simulink model "model1"  (R2021b)
settings: Solver=VariableStepAuto  StartTime=0.0  StopTime=10.0  FixedStep=0.001  RelTol=1e-3
undefined symbols (not defined in the file): Newton, Raphson
libraries: simulink x21, slpidlib x7
(part 1 of 2)
settings Model: Creator=O  LastModifiedBy=wangzixuan

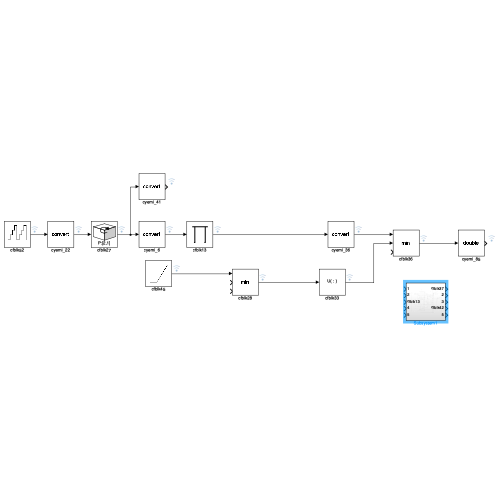
[thumbnail: Simulink's stored preview of the top-level diagram]
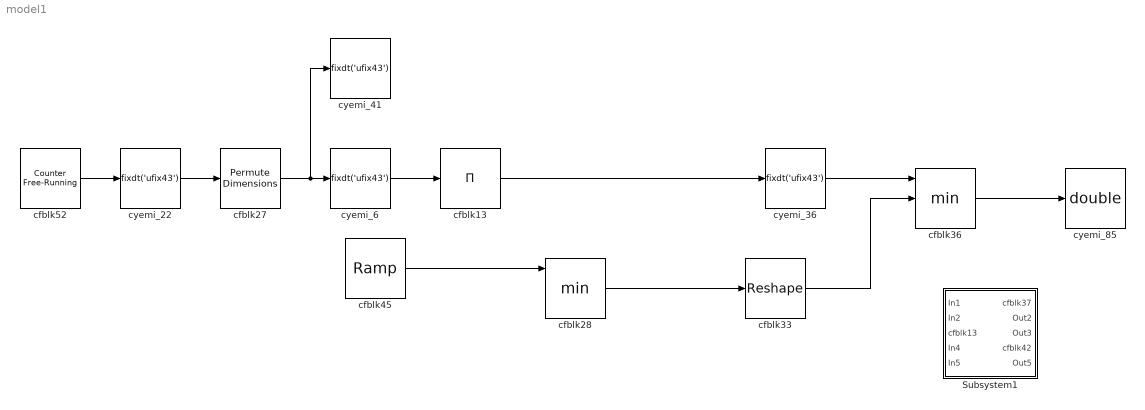
== system model1 ==
  Subsystem1 : Subsystem
  cfblk13 : Product  Inputs=*  OutDataTypeStr=fixdt('ufix43')
  cfblk27 : PermuteDimensions
  cfblk28 : MinMax  Inputs=3  OutDataTypeStr=double
  cfblk33 : Reshape
  cfblk36 : MinMax  Inputs=3  OutDataTypeStr=double
  cfblk45 : simulink/Sources/Ramp  slope=[2140.187855]  start=[6.196724]  InitialOutput=[541750.410278]
  cfblk52 : simulink/Sources/Counter Free-Running  NumBits=[43.000000]  tsamp=1
  cyemi_{6,22,36,41} (4 alike) : DataTypeConversion  OutDataTypeStr=fixdt('ufix43')
  cyemi_85 : DataTypeConversion  OutDataTypeStr=double
  wires:
  cfblk27/1 -> cyemi_41/1, cyemi_6/1
  cfblk52/1 -> cyemi_22/1
  cfblk33/1 -> cfblk36/2
  cyemi_36/1 -> cfblk36/1
  cfblk45/1 -> cfblk28/1
  cfblk36/1 -> cyemi_85/1
  cfblk28/1 -> cfblk33/1
  cyemi_6/1 -> cfblk13/1
  cfblk13/1 -> cyemi_36/1
  cyemi_22/1 -> cfblk27/1

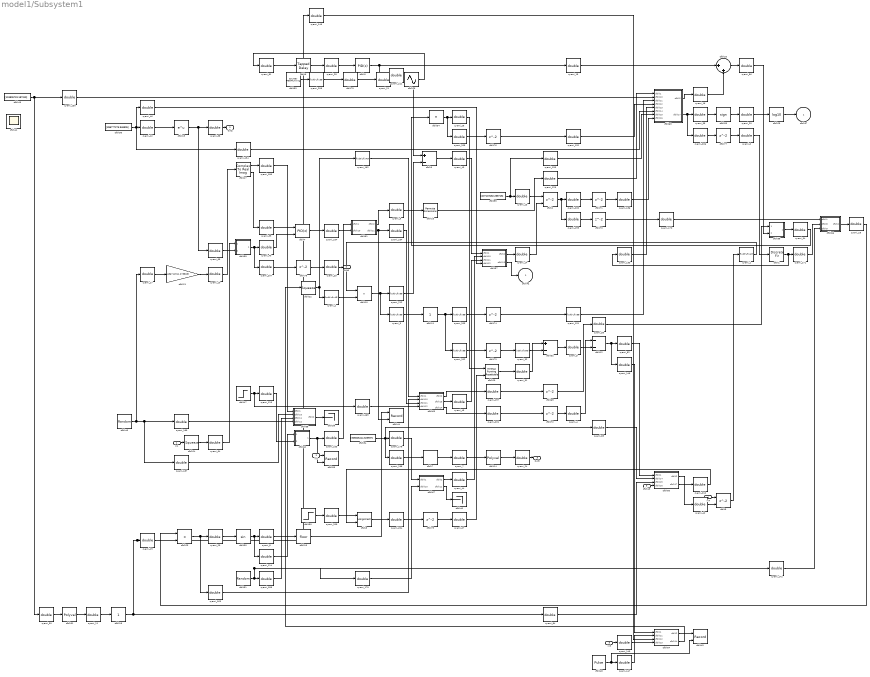
== system model1/Subsystem1 ==
  In1 : Inport
  In2 : Inport  Port=2
  cfblk13 : Inport  Port=3
  In4 : Inport  Port=4
  In5 : Inport  Port=5
  cfblk1 : DiscreteFir  SampleTime=1
  cfblk10 : DotProduct  OutDataTypeStr=fixdt('ufix86')  InputSameDT=on
  cfblk11 : simulink/Math Operations/Slider Gain  gain=1  low=0  high=2
  cfblk12 : Sum  Inputs=--  OutDataTypeStr=double
  cfblk14 : Polyval  Coefs=[ +2.081618890e-019, -1.441693666e-014, +4.719686976e-010, -8.536869453e-006, +1.621573104e-001, -8.087801117e+001 ]
  cfblk15 : Rounding
  cfblk16 : PermuteDimensions
  cfblk17 : ComplexToRealImag
  cfblk18 : simulink/Math Operations/Slider Gain  gain=1  low=0  high=2
  cfblk19 : Math  OutDataTypeStr=double  SaturateOnIntegerOverflow=on
  cfblk2 : Delay  ShowEnablePort=on  SampleTime=1
      settings: InputPortMap=u0,e6
  cfblk20 : Sum  Inputs=|++  OutDataTypeStr=double
  cfblk21 : Gain  Gain=[486711511.278808]  OutDataTypeStr=double
  cfblk22 : Squeeze
  cfblk23 : Product  OutDataTypeStr=double
  cfblk24 : Squeeze
  cfblk25 : Math  Operator=log10  OutDataTypeStr=double  SaturateOnIntegerOverflow=on
  cfblk26 : Sin  TimeSource=Use external signal  SampleTime=0
  cfblk29 : simulink/Math Operations/MinMax Running Resettable  Function=min  vinit=0.0
  cfblk3 : slpidlib/PID Controller  Controller=PID  Form=Parallel  TimeDomain=Discrete-time  UseExternalTs=off  SampleTime=1  IntegratorMethod=Forward Euler  FilterMethod=Forward Euler  ControllerParametersSource=internal  P=1  I=1  D=0  UseFilter=on  N=100  TunerSelectOption=Transfer Function Based (PID Tuner App)  InitialConditionSource=internal  InitialConditionForIntegrator=0  InitialConditionForFilter=0  DifferentiatorICPrevScaledInput=0  ExternalReset=none  TrackingMode=off  Kt=1  LimitOutput=off  SatLimitsSource=internal  UpperSaturationLimit=inf  LowerSaturationLimit=-inf  LinearizeAsGain=off  AntiWindupMode=none  Kb=1  POutMin=[]  POutMax=[]  IOutMin=[]  IOutMax=[]  DOutMin=[]  DOutMax=[]  NOutMin=[]  NOutMax=[]  SumOutMin=[]  SumOutMax=[]  SaturationOutMin=[]  SaturationOutMax=[]  PParamMin=[]  PParamMax=[]  IParamMin=[]  IParamMax=[]  DParamMin=[]  DParamMax=[]  NParamMin=[]  NParamMax=[]  KbParamMin=[]  KbParamMax=[]  KtParamMin=[]  KtParamMax=[]  KbOutMin=[]  KbOutMax=[]  KtOutMin=[]  KtOutMax=[]  IntegratorOutMin=[]  IntegratorOutMax=[]  FilterOutMin=[]  FilterOutMax=[]  SumI1OutMin=[]  SumI1OutMax=[]  SumI2OutMin=[]  SumI2OutMax=[]  SumI3OutMin=[]  SumI3OutMax=[]  SumI4OutMin=[]  SumI4OutMax=[]  SumDOutMin=[]  SumDOutMax=[]  DifferentiatorOutMin=[]  DifferentiatorOutMax=[]  FilterDiffOutCoefMin=[]  FilterDiffOutCoefMax=[]  ReciprocalOutMin=[]  ReciprocalOutMax=[]  SumDenOutMin=[]  SumDenOutMax=[]  SumNumOutMin=[]  SumNumOutMax=[]  DivideOutMin=[]  DivideOutMax=[]  UdiffTsProdOutMin=[]  UdiffTsProdOutMax=[]  NTsProdOutMin=[]  NTsProdOutMax=[]  UintegralTsProdOutMin=[]  UintegralTsProdOutMax=[]  UngainTsProdOutMin=[]  UngainTsProdOutMax=[]  IntegratorContinuousStateAttributes=''  IntegratorStateMustResolveToSignalObject=off  IntegratorRTWStateStorageClass=Auto  FilterContinuousStateAttributes=''  FilterStateMustResolveToSignalObject=off  FilterRTWStateStorageClass=Auto  ParallelPVariant=InternalParameters  IdealPVariant=Disabled  IVariant=InternalParameters  DVariant=InternalParameters  IntegratorVariant=Discrete  SatVariant=Disabled  AWVariant=Passthrough  PCopyVariant=Disabled  TRVariant=Disabled  FdbkBlocksVariant=Forward  IdealPFdbkVariant=Disabled  SatFdbkVariant=Disabled  DerivativeFilterVariant=ForwardEulerFilter  NVariant=InternalParameters  NCopyVariant=Disabled  FilterICVariant=InternalICsFilter  IntegratorICVariant=InternalICs  ExternalResetVariant=Disabled  TRSumVariant=Passthrough  SumFdbkVariant=Disabled  SumVariant=Sum_PID  TsampFilterVariant=InternalTs  TsampNgainVariant=Passthrough  TsampIntegralVariant=Passthrough  ExternalSaturationOutDataTypeStr=Inherit: Same as second input
  cfblk30 : Trigonometry
  cfblk31 : Polyval  Coefs=[ +2.081618890e-019, -1.441693666e-014, +4.719686976e-010, -8.536869453e-006, +1.621573104e-001, -8.087801117e+001 ]
  cfblk32 : Sum  Inputs=+-  OutDataTypeStr=double
  cfblk34 : Product  Inputs=*  OutDataTypeStr=double
  cfblk35 : Signum
  cfblk38 : Record  FileSettingsInternal="{\"entries\":[{\"content\":{\"excelSettings\":{\"content\":{},\"type\":\"Streamout.ExcelSettings\"}},\"type\":\"Streamout.FileSettingStorage\",\"uuid\":\"557034d7-062e-42b8-a2bb-f1e2b1ffd268\"}],\"packageUris\":[\"http://schema.mathworks.com/mf0/streamout_blocks/R2020a\"],\"version\":\"1.0\"}"  Layout=[1 1]  SignalsInternal="{\"entries\":[{\"content\":{\"signals\":[{\"content\":{\"blockPath\":[\"model1/Subsystem1/cfblk38\"],\"channel\":[],\"dimensions\":[1],\"domain\":\"model1/Subsystem1/cfblk38\",\"lineColor\":\"#ff6929\",\"plots\":[],\"port\":2,\"sid\":[\"\"],\"signalID\":318,\"signalName\":\"cfblk62\"},\"type\":\"RecordBlkView.Signal\",\"uuid\":\"ab7d02b3-7a9e-4b65-9ebb-9438a1fcbe7d\"},{\"content\":{\"blockPath\":[\"model1/Subsystem1/cfblk38\"],\"channel\":[],\"dimensions\":[1],\"domain\":\"model1/Subsystem1/cfblk38\",\"lineColor\":\"#ff13a6\",\"plots\":[],\"port\":1,\"sid\":[\"\"],\"signalID\":386,\"signalName\":\"In2\"},\"type\":\"RecordBlkView.Signal\",\"uuid\":\"c1cead91-3119-44b1-8a04-6ec5df58031d\"}]},\"type\":\"RecordBlkView.InputSignals\",\"uuid\":\"4d33e7d7-37c6-4ab8-bb5d-a37d3effe30e\"}],\"packageUris\":[\"http://schema.mathworks.com/mf0/streamout_blocks/R2020a\"],\"version\":\"1.0\"}"  VisualizationBindings="{\"xyplotplugin\":{\"info\":[{\"series\":[],\"subplotID\":1}]}}"  CompatibilityTag=XY
  cfblk39 : Terminator
  cfblk4 : slpidlib/PID Controller (2DOF)  Controller=PID  Form=Parallel  TimeDomain=Discrete-time  UseExternalTs=off  SampleTime=1  IntegratorMethod=Forward Euler  FilterMethod=Forward Euler  ControllerParametersSource=internal  P=1  I=1  D=0  UseFilter=on  N=100  b=1  c=1  TunerSelectOption=Transfer Function Based (PID Tuner App)  InitialConditionSource=internal  InitialConditionForIntegrator=0  InitialConditionForFilter=0  DifferentiatorICPrevScaledInput=0  ExternalReset=none  TrackingMode=off  Kt=1  LimitOutput=off  SatLimitsSource=internal  UpperSaturationLimit=inf  LowerSaturationLimit=-inf  LinearizeAsGain=off  AntiWindupMode=none  Kb=1  POutMin=[]  POutMax=[]  IOutMin=[]  IOutMax=[]  DOutMin=[]  DOutMax=[]  NOutMin=[]  NOutMax=[]  bOutMin=[]  bOutMax=[]  cOutMin=[]  cOutMax=[]  SumOutMin=[]  SumOutMax=[]  SaturationOutMin=[]  SaturationOutMax=[]  PParamMin=[]  PParamMax=[]  IParamMin=[]  IParamMax=[]  DParamMin=[]  DParamMax=[]  NParamMin=[]  NParamMax=[]  bParamMin=[]  bParamMax=[]  cParamMin=[]  cParamMax=[]  KbParamMin=[]  KbParamMax=[]  KtParamMin=[]  KtParamMax=[]  KbOutMin=[]  KbOutMax=[]  KtOutMin=[]  KtOutMax=[]  IntegratorOutMin=[]  IntegratorOutMax=[]  FilterOutMin=[]  FilterOutMax=[]  SumI1OutMin=[]  SumI1OutMax=[]  SumI2OutMin=[]  SumI2OutMax=[]  SumI3OutMin=[]  SumI3OutMax=[]  SumI4OutMin=[]  SumI4OutMax=[]  SumDOutMin=[]  SumDOutMax=[]  Sum1OutMin=[]  Sum1OutMax=[]  Sum2OutMin=[]  Sum2OutMax=[]  Sum3OutMin=[]  Sum3OutMax=[]  DifferentiatorOutMin=[]  DifferentiatorOutMax=[]  FilterDiffOutCoefMin=[]  FilterDiffOutCoefMax=[]  ReciprocalOutMin=[]  ReciprocalOutMax=[]  SumDenOutMin=[]  SumDenOutMax=[]  SumNumOutMin=[]  SumNumOutMax=[]  DivideOutMin=[]  DivideOutMax=[]  UdiffTsProdOutMin=[]  UdiffTsProdOutMax=[]  NTsProdOutMin=[]  NTsProdOutMax=[]  UintegralTsProdOutMin=[]  UintegralTsProdOutMax=[]  UngainTsProdOutMin=[]  UngainTsProdOutMax=[]  IntegratorContinuousStateAttributes=''  IntegratorStateMustResolveToSignalObject=off  IntegratorRTWStateStorageClass=Auto  FilterContinuousStateAttributes=''  FilterStateMustResolveToSignalObject=off  FilterRTWStateStorageClass=Auto  ParallelPVariant=InternalParameters  IdealPVariant=Disabled  IVariant=InternalParameters  DVariant=InternalParameters  bVariant=InternalParameters  cVariant=InternalParameters  IntegratorVariant=Discrete  SatVariant=Disabled  AWVariant=Passthrough  PCopyVariant=Disabled  TRVariant=Disabled  FdbkBlocksVariant=Forward  IdealPFdbkVariant=Disabled  SatFdbkVariant=Disabled  DerivativeFilterVariant=ForwardEulerFilter  NVariant=InternalParameters  NCopyVariant=Disabled  FilterICVariant=InternalICsFilter  IntegratorICVariant=InternalICs  ExternalResetVariant=Disabled  TRSumVariant=Passthrough  SumFdbkVariant=Disabled  SumVariant=Sum_PID  TsampFilterVariant=InternalTs  TsampNgainVariant=Passthrough  TsampIntegralVariant=Passthrough  ExternalSaturationOutDataTypeStr=Inherit: Same as second input
      settings: SourceProductBaseCode=SL
  cfblk40 : Terminator
  cfblk41 : Scope
      settings: Floating=on
  cfblk43 : Record  FileSettingsInternal="{\"entries\":[{\"content\":{\"excelSettings\":{\"content\":{},\"type\":\"Streamout.ExcelSettings\"}},\"type\":\"Streamout.FileSettingStorage\",\"uuid\":\"05afdac6-b020-49f8-8b8c-a1ffa4635084\"}],\"packageUris\":[\"http://schema.mathworks.com/mf0/streamout_blocks/R2020a\"],\"version\":\"1.0\"}"  Layout=[1 1]  SignalsInternal="{\"entries\":[{\"content\":{\"signals\":[{\"content\":{\"blockPath\":[\"model1/Subsystem1/cfblk43\"],\"channel\":[],\"dimensions\":[1],\"domain\":\"model1/Subsystem1/cfblk43\",\"lineColor\":\"#b746ff\",\"plots\":[],\"port\":1,\"sid\":[\"\"],\"signalID\":322,\"signalName\":\"cfblk64:1\"},\"type\":\"RecordBlkView.Signal\",\"uuid\":\"b89210de-1096-4b1a-b254-886097bf9b24\"},{\"content\":{\"blockPath\":[\"model1/Subsystem1/cfblk43\"],\"channel\":[],\"dimensions\":[1],\"domain\":\"model1/Subsystem1/cfblk43\",\"lineColor\":\"#64d413\",\"plots\":[],\"port\":2,\"sid\":[\"\"],\"signalID\":326,\"signalName\":\"cfblk48\"},\"type\":\"RecordBlkView.Signal\",\"uuid\":\"c775b4e3-5fa6-4147-9682-4ab041113417\"}]},\"type\":\"RecordBlkView.InputSignals\",\"uuid\":\"8fc3c609-e7c6-4487-a5b8-ce75645389d4\"}],\"packageUris\":[\"http://schema.mathworks.com/mf0/streamout_blocks/R2020a\"],\"version\":\"1.0\"}"  VisualizationBindings="{\"xyplotplugin\":{\"info\":[{\"series\":[],\"subplotID\":1}]}}"  CompatibilityTag=XY
  cfblk44 : Record  FileSettingsInternal="{\"entries\":[{\"content\":{\"excelSettings\":{\"content\":{},\"type\":\"Streamout.ExcelSettings\"}},\"type\":\"Streamout.FileSettingStorage\",\"uuid\":\"f2e21b0c-007e-424c-9b78-7cb041026585\"}],\"packageUris\":[\"http://schema.mathworks.com/mf0/streamout_blocks/R2020a\"],\"version\":\"1.0\"}"  Layout=[1 1]  SignalsInternal="{\"entries\":[{\"content\":{\"signals\":[{\"content\":{\"blockPath\":[\"model1/Subsystem1/cfblk44\"],\"channel\":[],\"dimensions\":[1],\"domain\":\"model1/Subsystem1/cfblk44\",\"lineColor\":\"#ff13a6\",\"plots\":[],\"port\":1,\"sid\":[\"\"],\"signalID\":330,\"signalName\":\"cfblk15\"},\"type\":\"RecordBlkView.Signal\",\"uuid\":\"5d98a457-5196-4a25-837c-2ae2c00d410e\"},{\"content\":{\"blockPath\":[\"model1/Subsystem1/cfblk44\"],\"channel\":[],\"dimensions\":[1],\"domain\":\"model1/Subsystem1/cfblk44\",\"lineColor\":\"#fe330a\",\"plots\":[],\"port\":2,\"sid\":[\"\"],\"signalID\":334,\"signalName\":\"cfblk61:2\"},\"type\":\"RecordBlkView.Signal\",\"uuid\":\"37265b59-f577-41b0-b9ae-f6129d80ff15\"}]},\"type\":\"RecordBlkView.InputSignals\",\"uuid\":\"38bcc02e-858f-4c58-a572-d2fc91423907\"}],\"packageUris\":[\"http://schema.mathworks.com/mf0/streamout_blocks/R2020a\"],\"version\":\"1.0\"}"  VisualizationBindings="{\"xyplotplugin\":{\"info\":[{\"series\":[],\"subplotID\":1}]}}"  CompatibilityTag=XY
  cfblk46 : RandomNumber  Mean=[99195.516790]  Variance=[63142.809470]  Seed=[502694250.000000]  SampleTime=0.1
  cfblk47 : Step  Time=[40.000000]  Before=[-902205539.762799]  After=[431875218.013777]  SampleTime=0
  cfblk48 : DiscretePulseGenerator  PulseType=Time based  Amplitude=[-808136407.788434]  Period=[60696491.639829]  PulseWidth=5  PhaseDelay=[4.000000]
  cfblk49 : Constant  Value=[119805723.187319]  OutDataTypeStr=double  SampleTime=1
  cfblk5 : Delay  ShowEnablePort=on  SampleTime=1
      settings: InputPortMap=u0,e6
  cfblk50 : Step  Time=[14.000000]  Before=[438737412.518362]  After=[-271082864.971538]  SampleTime=0
  cfblk51 : UniformRandomNumber  Minimum=[-8048498288.843409]  Maximum=[1672685997.545453]  Seed=[83431266.000000]  SampleTime=0.1
  cfblk53 : simulink/Sources/Counter Free-Running  NumBits=[39.000000]  tsamp=1
  cfblk54 : Constant  Value=[306626414.325937]  OutDataTypeStr=double  SampleTime=1
  cfblk55 : Constant  Value=[207119182.268716]  OutDataTypeStr=double  SampleTime=1
  cfblk56 : Constant  Value=[396777275.946905]  OutDataTypeStr=double  SampleTime=1
  cfblk57 : Subsystem
  cfblk58 : Subsystem
  cfblk59 : Subsystem
  cfblk6 : simulink/Discrete/Tapped Delay  vinit=0.0  samptime=-1  NumDelays=1  DelayOrder=Oldest  includeCurrent=off
  cfblk60 : Subsystem
  cfblk61 : Subsystem
  cfblk62 : Subsystem
  cfblk63 : Subsystem
  cfblk64 : Subsystem
  cfblk65 : Subsystem
  cfblk66 : Subsystem
  cfblk67 : Subsystem
  cfblk68 : Subsystem
  cfblk{69..78} (10 alike) : Delay  SampleTime=1
  cfblk7 : DiscreteStateSpace
  cfblk79 : DataTypeConversion  OutDataTypeStr=double
  cfblk8 : Assignment  DiagnosticForDimensions=Warning  IndexOptions=Index vector (dialog)  Indices=1  OutputSizes=1
  cfblk9 : Sum  Inputs=+-  OutDataTypeStr=double
  cyemi_{0,4..5,7..21,24..31,34..35,38..40,42..46,55..56,64..65,81..84,103..104,114..115,129..130,132..136,146..149,163..165,170..172,178..179,186..189,197..201,204..207,209..211} (83 alike) : DataTypeConversion  OutDataTypeStr=double
  cyemi_1 : DataTypeConversion  OutDataTypeStr=fixdt('ufix43')
  cyemi_{3,32,131,202..203,212} (6 alike) : DataTypeConversion  OutDataTypeStr=fixdt('ufix86')
  cyemi_162 : DataTypeConversion  OutDataTypeStr=fixdt('ufix43')
  cyemi_2 : DataTypeConversion  OutDataTypeStr=fixdt('ufix43')
  cyemi_208 : DataTypeConversion  OutDataTypeStr=fixdt('ufix39')
  cfblk37 : Outport
  Out2 : Outport  Port=2
  Out3 : Outport  Port=3
  cfblk42 : Outport  Port=4
  Out5 : Outport  Port=5
  wires:
  cyemi_162/1 -> cfblk65/1(cfblk1)
  cyemi_43/1 -> cfblk57/1(cfblk1)
  cyemi_9/1 -> cfblk16/1
  cyemi_20/1 -> cfblk25/1
  cfblk67/2(cfblk11) -> cfblk40/1
  cyemi_198/1 -> cfblk7/1
  cyemi_83/1 -> cfblk60/2(cfblk14)
  cyemi_81/1 -> cfblk6/1
  cfblk64/2(cfblk14) -> cfblk22/1
  cfblk6/1 -> cyemi_28/1
  cyemi_15/1 -> cfblk20/1
  cyemi_172/1 -> cfblk66/3(cfblk9)
  cfblk78/1 -> cyemi_25/1
  cyemi_31/1 -> cfblk32/1
  cyemi_208/1 -> cfblk79/1
  cyemi_45/1 -> cfblk57/3(cfblk11)
  cyemi_114/1 -> cfblk62/1(cfblk1)
  cyemi_28/1 -> cfblk3/1
  cfblk5/1 -> cyemi_1/1
  cyemi_4/1 -> cfblk12/1
  cfblk25/1 -> cfblk37/1
  cfblk30/1 -> cyemi_114/1, cyemi_8/1
  cyemi_212/1 -> cfblk9/2
  cyemi_7/1 -> cfblk14/1
  cyemi_0/1 -> cfblk1/1
  cyemi_131/1 -> cfblk63/3(cfblk11)
  cyemi_26/1 -> cfblk29/1
  cfblk58/1(cfblk2) -> cyemi_34/1
  cyemi_197/1 -> cfblk69/1
  cyemi_135/1 -> cfblk63/7(cfblk15)
  cfblk71/1 -> cyemi_136/1
  cyemi_40/1 -> cfblk4/2
  cyemi_46/1 -> cfblk57/4(cfblk12)
  cfblk7/1 -> cyemi_7/1
  cyemi_5/1 -> cfblk12/2
  cyemi_17/1 -> cfblk21/1
  cyemi_13/1 -> cfblk2/1
  cyemi_207/1 -> cfblk78/1
  cyemi_39/1 -> cfblk4/1
  cyemi_202/1 -> cfblk73/1
  cfblk4/1 -> cyemi_104/1
  cyemi_18/1 -> cfblk23/1
  cyemi_3/1 -> cfblk11/1
  cyemi_136/1 -> cfblk63/8(cfblk16)
  cfblk68/1(cfblk2) -> cfblk39/1
  cyemi_21/1 -> cfblk26/1
  cfblk16/1 -> cyemi_129/1
  cfblk75/1 -> cyemi_27/1
  cfblk76/1 -> cyemi_132/1
  cyemi_148/1 -> cfblk64/3(cfblk12)
  cfblk1/1 -> cyemi_171/1, cyemi_133/1
  cfblk15/1 -> cfblk44/1
  cyemi_34/1 -> cfblk34/1
  cyemi_201/1 -> cfblk72/1
  cyemi_82/1 -> cfblk60/1(cfblk1)
  cyemi_146/1 -> cfblk64/1(cfblk1)
  cfblk66/1(cfblk2) -> cyemi_18/1
  cfblk61/1(cfblk2) -> cyemi_9/1
  cyemi_186/1 -> cfblk68/1(cfblk1)
  cyemi_38/1 -> Out2/1
  cyemi_104/1 -> cfblk61/2(cfblk10)
  cyemi_84/1 -> cfblk60/3(cfblk15)
  cyemi_203/1 -> cfblk74/1
  cyemi_129/1 -> cfblk63/1(cfblk1)
  cfblk59/1(cfblk2) -> cyemi_207/1, cyemi_40/1
  cfblk9/1 -> cyemi_43/1
  cfblk69/1 -> cyemi_55/1
  cfblk65/2(cfblk13) -> cyemi_45/1
  cyemi_130/1 -> cfblk63/2(cfblk10)
  cyemi_11/1 -> cfblk18/1
  cyemi_56/1 -> cfblk58/2(cfblk8)
  cfblk2/1 -> cyemi_200/1, cyemi_199/1
  cfblk14/1 -> cyemi_24/1
  cfblk74/1 -> cyemi_131/1
  cfblk46/1 -> cyemi_189/1, cyemi_187/1, cyemi_17/1
  cfblk63/2(cfblk17) -> cyemi_206/1, cyemi_35/1
  cfblk70/1 -> cyemi_170/1
  cfblk79/1 -> cyemi_21/1
  cyemi_205/1 -> cfblk76/1
  cfblk11/1 -> cyemi_203/1, cyemi_202/1
  cyemi_206/1 -> cfblk77/1
  cfblk72/1 -> cyemi_4/1
  cfblk26/1 -> cyemi_81/1
  cfblk64/1(cfblk2) -> cfblk43/1
  cyemi_32/1 -> cfblk32/2
  cyemi_199/1 -> cfblk70/1
  cyemi_25/1 -> Out3/1
  cfblk57/2(cfblk13) -> cfblk42/1
  cfblk67/1(cfblk2) -> cyemi_44/1
  cyemi_164/1 -> cfblk65/3(cfblk11)
  cyemi_64/1 -> cfblk59/1(cfblk1)
  cfblk22/1 -> cyemi_162/1, cyemi_2/1
  cfblk3/1 -> cyemi_211/1, cyemi_15/1
  cyemi_179/1 -> cfblk67/2(cfblk10)
  cfblk24/1 -> cyemi_64/1
  In5/1 -> cyemi_149/1
  cyemi_133/1 -> cfblk63/5(cfblk13)
  cyemi_19/1 -> cfblk23/2
  cfblk60/1(cfblk2) -> cyemi_42/1
  cfblk20/1 -> cyemi_56/1
  cyemi_189/1 -> cfblk68/4(cfblk12)
  cfblk77/1 -> cyemi_0/1
  cyemi_65/1 -> cfblk59/2(cfblk16)
  cyemi_147/1 -> cfblk64/2(cfblk11)
  cfblk55/1 -> cyemi_135/1, cyemi_13/1
  cyemi_115/1 -> cfblk62/2(cfblk12)
  cyemi_10/1 -> cfblk17/1
  cfblk60/2(cfblk17) -> cyemi_210/1
  cfblk29/1 -> cyemi_31/1
  cyemi_27/1 -> cfblk29/2
  cfblk49/1 -> cyemi_130/1, cyemi_30/1
  In1/1 -> cfblk24/1
  cyemi_188/1 -> cfblk68/3(cfblk11)
  cfblk73/1 -> cyemi_32/1
  cfblk54/1 -> cyemi_178/1, cyemi_83/1, cyemi_198/1
  cyemi_209/1 -> cfblk8/1
  cfblk56/1 -> cyemi_46/1, cyemi_134/1, cyemi_12/1
  cyemi_210/1 -> cfblk8/2
  cyemi_103/1 -> cfblk61/1(cfblk1)
  cyemi_16/1 -> cfblk20/2
  In2/1 -> cfblk38/1
  cyemi_171/1 -> cfblk66/2(cfblk8)
  cyemi_44/1 -> cfblk57/2(cfblk10)
  cyemi_134/1 -> cfblk63/6(cfblk14)
  cyemi_24/1 -> Out5/1
  cyemi_30/1 -> cfblk31/1
  cyemi_2/1 -> cfblk10/2
  cfblk63/1(cfblk2) -> cyemi_16/1
  cfblk17/1 -> cyemi_186/1
  cfblk47/1 -> cyemi_165/1, cyemi_115/1
  cyemi_132/1 -> cfblk63/4(cfblk12)
  cfblk32/1 -> cyemi_5/1
  cyemi_8/1 -> cfblk15/1
  cyemi_163/1 -> cfblk65/2(cfblk10)
  cfblk65/3(cfblk14) -> cyemi_201/1
  cyemi_149/1 -> cfblk64/4(cfblk13)
  cyemi_200/1 -> cfblk71/1
  cfblk13/1 -> cfblk60/4(cfblk16)
  In4/1 -> cfblk5/1
  cfblk62/1(cfblk2) -> cyemi_103/1, cfblk38/2
  cfblk34/1 -> cyemi_205/1, cyemi_26/1
  cfblk61/2(cfblk11) -> cyemi_164/1, cfblk44/2
  cfblk21/1 -> cyemi_10/1
  cfblk53/1 -> cyemi_208/1
  cfblk50/1 -> cyemi_209/1
  cfblk23/1 -> cyemi_163/1, cyemi_29/1
  cfblk31/1 -> cyemi_11/1
  cyemi_42/1 -> cfblk5/2
  cyemi_12/1 -> cfblk19/1
  cyemi_29/1 -> cfblk30/1
  cfblk48/1 -> cyemi_147/1, cfblk43/2
  cfblk19/1 -> cyemi_65/1, cyemi_38/1
  cfblk12/1 -> cyemi_146/1, cyemi_82/1
  cfblk51/1 -> cyemi_172/1, cyemi_179/1, cyemi_188/1
  cfblk17/2 -> cyemi_39/1
  cyemi_204/1 -> cfblk75/1
  cyemi_14/1 -> cfblk2/2
  cfblk8/1 -> cyemi_204/1
  cyemi_1/1 -> cfblk10/1
  cyemi_165/1 -> cfblk65/4(cfblk12)
  cyemi_35/1 -> cfblk35/1
  cfblk35/1 -> cyemi_20/1
  cyemi_55/1 -> cfblk58/1(cfblk1)
  cyemi_187/1 -> cfblk68/2(cfblk10)
  cfblk10/1 -> cyemi_212/1, cyemi_3/1
  cfblk57/1(cfblk2) -> cyemi_14/1
  cfblk65/1(cfblk2) -> cyemi_197/1
  cyemi_211/1 -> cfblk9/1
  cfblk18/1 -> cyemi_148/1, cyemi_19/1, cyemi_84/1
  cyemi_178/1 -> cfblk67/1(cfblk1)
  cyemi_170/1 -> cfblk66/1(cfblk1)

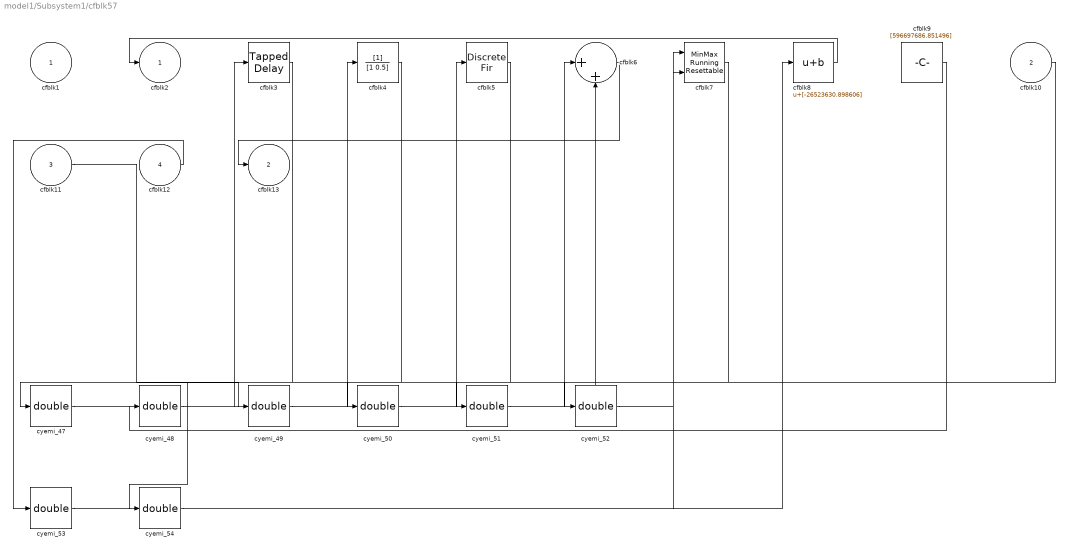
== system model1/Subsystem1/cfblk57 ==
  cfblk1 : Inport
  cfblk10 : Inport  Port=2
  cfblk11 : Inport  Port=3
  cfblk12 : Inport  Port=4
  cfblk3 : simulink/Discrete/Tapped Delay  vinit=0.0  samptime=-1  NumDelays=1  DelayOrder=Oldest  includeCurrent=off
  cfblk4 : DiscreteFilter  SampleTime=1
  cfblk5 : DiscreteFir  SampleTime=1
  cfblk6 : Sum  Inputs=|++  OutDataTypeStr=double
  cfblk7 : simulink/Math Operations/MinMax Running Resettable  Function=min  vinit=0.0
  cfblk8 : Bias  Bias=[-26523630.898606]
  cfblk9 : Constant  Value=[596697686.851496]  OutDataTypeStr=double  SampleTime=1
  cyemi_{47..54} (8 alike) : DataTypeConversion  OutDataTypeStr=double
  cfblk2 : Outport
  cfblk13 : Outport  Port=2
  wires:
  cfblk6/1 -> cfblk13/1
  cfblk8/1 -> cfblk2/1
  cyemi_47/1 -> cfblk3/1
  cfblk5/1 -> cyemi_47/1
  cyemi_48/1 -> cfblk4/1
  cfblk9/1 -> cyemi_48/1
  cyemi_49/1 -> cfblk5/1
  cfblk11/1 -> cyemi_49/1
  cyemi_50/1 -> cfblk6/1
  cfblk4/1 -> cyemi_50/1
  cyemi_51/1 -> cfblk6/2
  cfblk7/1 -> cyemi_51/1
  cyemi_52/1 -> cfblk7/1
  cfblk10/1 -> cyemi_52/1
  cyemi_53/1 -> cfblk7/2
  cfblk12/1 -> cyemi_53/1
  cyemi_54/1 -> cfblk8/1
  cfblk3/1 -> cyemi_54/1

== system model1/Subsystem1/cfblk58 ==
  cfblk1 : Inport
  cfblk8 : Inport  Port=2
  cfblk3 : simulink/Discrete/Difference  ICPrevInput=0.0  OutMin=[]  OutMax=[]  OutDataTypeStr=double  OutputDataTypeScalingMode=double  OutDataType=fixdt(1, 16)  OutScaling=2^-10  DoSatur=off
  cfblk4 : DiscreteFir  SampleTime=1
  cfblk5 : UnaryMinus
  cfblk6 : Math  OutDataTypeStr=double  SaturateOnIntegerOverflow=on
  cfblk7 : Sum  Inputs=|++  OutDataTypeStr=double
  cfblk9 : Delay  SampleTime=1
  cyemi_{57..63} (7 alike) : DataTypeConversion  OutDataTypeStr=double
  cfblk2 : Outport
  wires:
  cfblk7/1 -> cfblk2/1
  cyemi_57/1 -> cfblk3/1
  cfblk8/1 -> cyemi_57/1
  cyemi_58/1 -> cfblk4/1
  cfblk9/1 -> cyemi_58/1
  cyemi_59/1 -> cfblk5/1
  cfblk4/1 -> cyemi_59/1
  cyemi_60/1 -> cfblk6/1
  cfblk3/1 -> cyemi_60/1
  cyemi_61/1 -> cfblk7/1
  cfblk6/1 -> cyemi_61/1
  cyemi_62/1 -> cfblk7/2
  cfblk1/1 -> cyemi_62/1
  cyemi_63/1 -> cfblk9/1
  cfblk5/1 -> cyemi_63/1

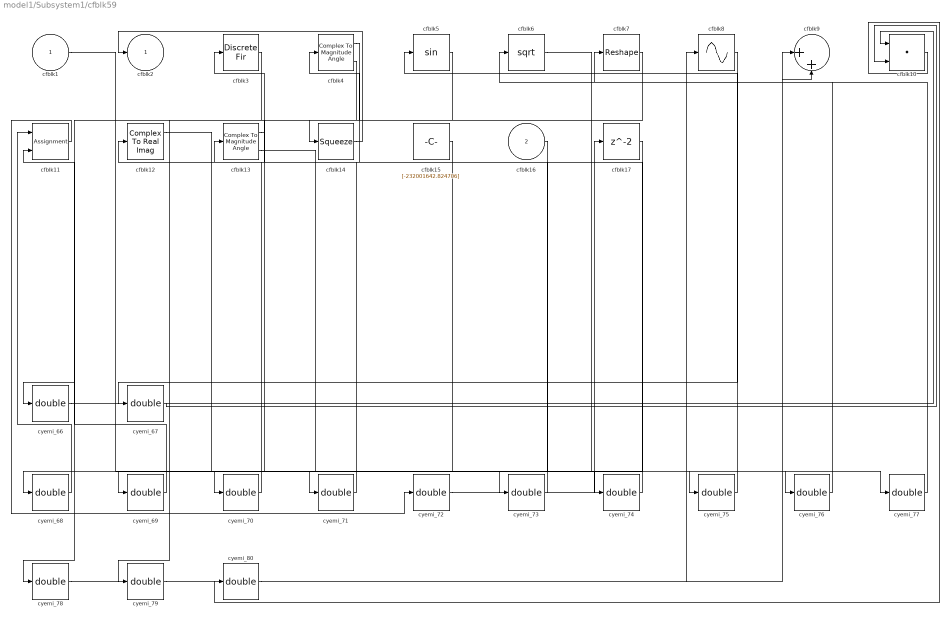
== system model1/Subsystem1/cfblk59 ==
  cfblk1 : Inport
  cfblk16 : Inport  Port=2
  cfblk10 : DotProduct  OutDataTypeStr=double  InputSameDT=on
  cfblk11 : Assignment  DiagnosticForDimensions=Warning  IndexOptions=Index vector (dialog)  Indices=1  OutputSizes=1
  cfblk12 : ComplexToRealImag
  cfblk13 : ComplexToMagnitudeAngle
  cfblk14 : Squeeze
  cfblk15 : Constant  Value=[-232001642.824706]  OutDataTypeStr=double  SampleTime=1
  cfblk17 : Delay  SampleTime=1
  cfblk3 : DiscreteFir  SampleTime=1
  cfblk4 : ComplexToMagnitudeAngle
  cfblk5 : Trigonometry
  cfblk6 : Sqrt  OutDataTypeStr=double  SaturateOnIntegerOverflow=on
  cfblk7 : Reshape
  cfblk8 : Sin  TimeSource=Use external signal  SampleTime=0
  cfblk9 : Sum  Inputs=|++  OutDataTypeStr=double
  cyemi_{66..80} (15 alike) : DataTypeConversion  OutDataTypeStr=double
  cfblk2 : Outport
  wires:
  cfblk4/1 -> cfblk14/1
  cfblk14/1 -> cfblk2/1
  cyemi_66/1 -> cfblk10/1
  cfblk4/2 -> cyemi_66/1
  cyemi_67/1 -> cfblk10/2
  cfblk8/1 -> cyemi_67/1
  cyemi_68/1 -> cfblk11/1
  cfblk3/1 -> cyemi_68/1
  cyemi_69/1 -> cfblk11/2
  cfblk13/1 -> cyemi_69/1
  cyemi_70/1 -> cfblk12/1
  cfblk7/1 -> cyemi_70/1
  cyemi_71/1 -> cfblk13/1
  cfblk15/1 -> cyemi_71/1
  cyemi_72/1 -> cfblk17/1
  cfblk11/1 -> cyemi_72/1
  cyemi_73/1 -> cfblk3/1
  cfblk17/1 -> cyemi_73/1
  cyemi_74/1 -> cfblk4/1
  cfblk1/1 -> cyemi_74/1
  cyemi_75/1 -> cfblk5/1
  cfblk12/1 -> cyemi_75/1
  cyemi_76/1 -> cfblk6/1
  cfblk13/2 -> cyemi_76/1
  cyemi_77/1 -> cfblk7/1
  cfblk6/1 -> cyemi_77/1
  cyemi_78/1 -> cfblk8/1
  cfblk16/1 -> cyemi_78/1
  cyemi_79/1 -> cfblk9/1
  cfblk5/1 -> cyemi_79/1
  cyemi_80/1 -> cfblk9/2
  cfblk10/1 -> cyemi_80/1

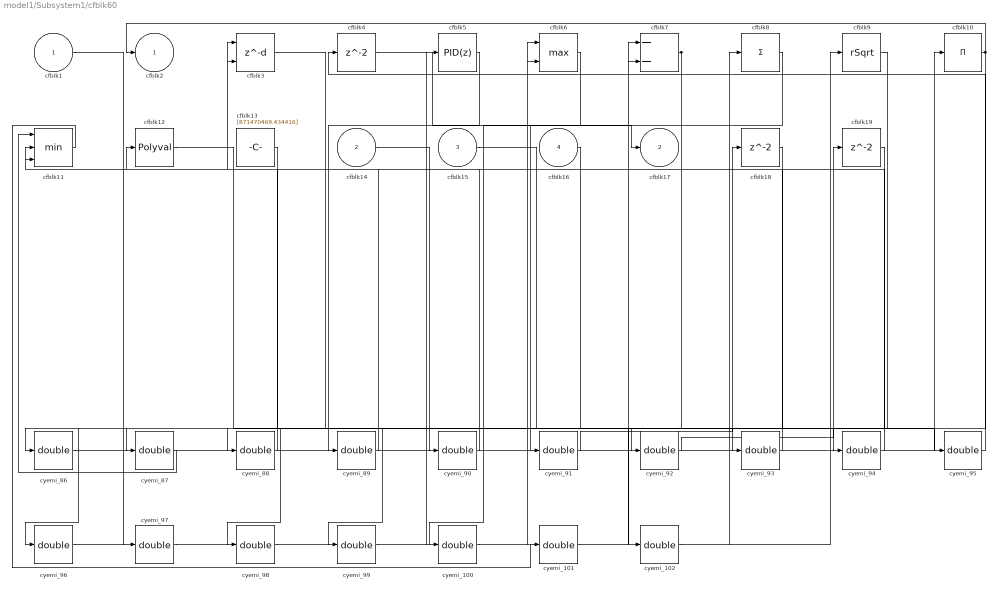
== system model1/Subsystem1/cfblk60 ==
  cfblk1 : Inport
  cfblk14 : Inport  Port=2
  cfblk15 : Inport  Port=3
  cfblk16 : Inport  Port=4
  cfblk10 : Product  Inputs=*  OutDataTypeStr=double
  cfblk11 : MinMax  Inputs=3  OutDataTypeStr=double
  cfblk12 : Polyval  Coefs=[ +2.081618890e-019, -1.441693666e-014, +4.719686976e-010, -8.536869453e-006, +1.621573104e-001, -8.087801117e+001 ]
  cfblk13 : Constant  Value=[871470469.434416]  OutDataTypeStr=double  SampleTime=1
  cfblk18 : Delay  SampleTime=1
  cfblk19 : Delay  SampleTime=1
  cfblk3 : Delay  DelayLengthSource=Input port  SampleTime=1
      settings: InputPortMap=u0,p1
  cfblk4 : Delay  SampleTime=1
  cfblk5 : slpidlib/PID Controller  Controller=PID  Form=Parallel  TimeDomain=Discrete-time  UseExternalTs=off  SampleTime=1  IntegratorMethod=Forward Euler  FilterMethod=Forward Euler  ControllerParametersSource=internal  P=1  I=1  D=0  UseFilter=on  N=100  TunerSelectOption=Transfer Function Based (PID Tuner App)  InitialConditionSource=internal  InitialConditionForIntegrator=0  InitialConditionForFilter=0  DifferentiatorICPrevScaledInput=0  ExternalReset=none  TrackingMode=off  Kt=1  LimitOutput=off  SatLimitsSource=internal  UpperSaturationLimit=inf  LowerSaturationLimit=-inf  LinearizeAsGain=off  AntiWindupMode=none  Kb=1  POutMin=[]  POutMax=[]  IOutMin=[]  IOutMax=[]  DOutMin=[]  DOutMax=[]  NOutMin=[]  NOutMax=[]  SumOutMin=[]  SumOutMax=[]  SaturationOutMin=[]  SaturationOutMax=[]  PParamMin=[]  PParamMax=[]  IParamMin=[]  IParamMax=[]  DParamMin=[]  DParamMax=[]  NParamMin=[]  NParamMax=[]  KbParamMin=[]  KbParamMax=[]  KtParamMin=[]  KtParamMax=[]  KbOutMin=[]  KbOutMax=[]  KtOutMin=[]  KtOutMax=[]  IntegratorOutMin=[]  IntegratorOutMax=[]  FilterOutMin=[]  FilterOutMax=[]  SumI1OutMin=[]  SumI1OutMax=[]  SumI2OutMin=[]  SumI2OutMax=[]  SumI3OutMin=[]  SumI3OutMax=[]  SumI4OutMin=[]  SumI4OutMax=[]  SumDOutMin=[]  SumDOutMax=[]  DifferentiatorOutMin=[]  DifferentiatorOutMax=[]  FilterDiffOutCoefMin=[]  FilterDiffOutCoefMax=[]  ReciprocalOutMin=[]  ReciprocalOutMax=[]  SumDenOutMin=[]  SumDenOutMax=[]  SumNumOutMin=[]  SumNumOutMax=[]  DivideOutMin=[]  DivideOutMax=[]  UdiffTsProdOutMin=[]  UdiffTsProdOutMax=[]  NTsProdOutMin=[]  NTsProdOutMax=[]  UintegralTsProdOutMin=[]  UintegralTsProdOutMax=[]  UngainTsProdOutMin=[]  UngainTsProdOutMax=[]  IntegratorContinuousStateAttributes=''  IntegratorStateMustResolveToSignalObject=off  IntegratorRTWStateStorageClass=Auto  FilterContinuousStateAttributes=''  FilterStateMustResolveToSignalObject=off  FilterRTWStateStorageClass=Auto  ParallelPVariant=InternalParameters  IdealPVariant=Disabled  IVariant=InternalParameters  DVariant=InternalParameters  IntegratorVariant=Discrete  SatVariant=Disabled  AWVariant=Passthrough  PCopyVariant=Disabled  TRVariant=Disabled  FdbkBlocksVariant=Forward  IdealPFdbkVariant=Disabled  SatFdbkVariant=Disabled  DerivativeFilterVariant=ForwardEulerFilter  NVariant=InternalParameters  NCopyVariant=Disabled  FilterICVariant=InternalICsFilter  IntegratorICVariant=InternalICs  ExternalResetVariant=Disabled  TRSumVariant=Passthrough  SumFdbkVariant=Disabled  SumVariant=Sum_PID  TsampFilterVariant=InternalTs  TsampNgainVariant=Passthrough  TsampIntegralVariant=Passthrough  ExternalSaturationOutDataTypeStr=Inherit: Same as second input
  cfblk6 : MinMax  Function=max  Inputs=2  OutDataTypeStr=double
  cfblk7 : Sum  Inputs=--  OutDataTypeStr=double
  cfblk8 : Sum  Inputs=+  OutDataTypeStr=double
  cfblk9 : Sqrt  Operator=rSqrt  OutDataTypeStr=double  AlgorithmType=Newton-Raphson  SaturateOnIntegerOverflow=on
  cyemi_{86..102} (17 alike) : DataTypeConversion  OutDataTypeStr=double
  cfblk2 : Outport
  cfblk17 : Outport  Port=2
  wires:
  cfblk7/1 -> cyemi_86/1, cyemi_92/1
  cfblk10/1 -> cfblk2/1, cyemi_96/1
  cfblk4/1 -> cfblk17/1
  cyemi_86/1 -> cfblk10/1
  cyemi_87/1 -> cfblk11/1
  cfblk13/1 -> cyemi_87/1
  cyemi_88/1 -> cfblk11/2
  cfblk16/1 -> cyemi_88/1
  cyemi_89/1 -> cfblk11/3
  cfblk5/1 -> cyemi_89/1
  cyemi_90/1 -> cfblk12/1
  cfblk14/1 -> cyemi_90/1
  cyemi_91/1 -> cfblk18/1
  cfblk8/1 -> cyemi_91/1
  cyemi_92/1 -> cfblk19/1
  cyemi_93/1 -> cfblk3/1
  cfblk15/1 -> cyemi_93/1
  cyemi_94/1 -> cfblk3/2
  cfblk9/1 -> cyemi_94/1
  cyemi_95/1 -> cfblk4/1
  cfblk3/1 -> cyemi_95/1
  cyemi_96/1 -> cfblk5/1
  cyemi_97/1 -> cfblk6/1
  cfblk1/1 -> cyemi_97/1
  cyemi_98/1 -> cfblk6/2
  cfblk19/1 -> cyemi_98/1
  cyemi_99/1 -> cfblk7/1
  cfblk18/1 -> cyemi_99/1
  cyemi_100/1 -> cfblk7/2
  cfblk6/1 -> cyemi_100/1
  cyemi_101/1 -> cfblk8/1
  cfblk11/1 -> cyemi_101/1
  cyemi_102/1 -> cfblk9/1
  cfblk12/1 -> cyemi_102/1

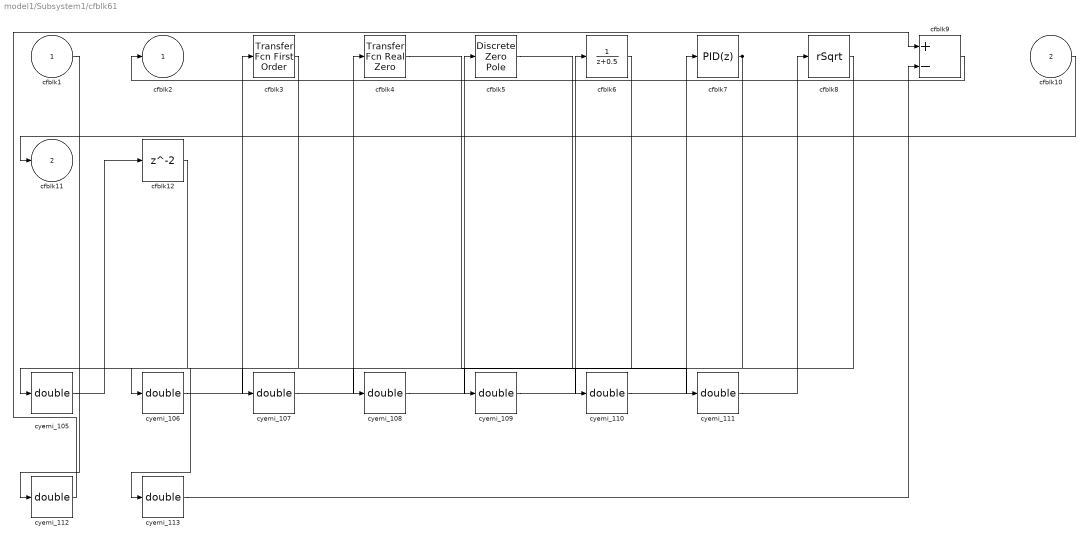
== system model1/Subsystem1/cfblk61 ==
  cfblk1 : Inport
  cfblk10 : Inport  Port=2
  cfblk12 : Delay  SampleTime=1
  cfblk3 : simulink/Discrete/Transfer Fcn First Order  PoleZ=0.95  ICPrevOutput=0.0  DoSatur=off
  cfblk4 : simulink/Discrete/Transfer Fcn Real Zero  ZeroZ=0.75  ICPrevInput=0.0  DoSatur=off
      settings: SourceProductBaseCode=SL
  cfblk5 : DiscreteZeroPole  Poles=[0 0.5]  Gain=1
  cfblk6 : DiscreteTransferFcn  SampleTime=1
  cfblk7 : slpidlib/PID Controller  Controller=PID  Form=Parallel  TimeDomain=Discrete-time  UseExternalTs=off  SampleTime=1  IntegratorMethod=Forward Euler  FilterMethod=Forward Euler  ControllerParametersSource=internal  P=1  I=1  D=0  UseFilter=on  N=100  TunerSelectOption=Transfer Function Based (PID Tuner App)  InitialConditionSource=internal  InitialConditionForIntegrator=0  InitialConditionForFilter=0  DifferentiatorICPrevScaledInput=0  ExternalReset=none  TrackingMode=off  Kt=1  LimitOutput=off  SatLimitsSource=internal  UpperSaturationLimit=inf  LowerSaturationLimit=-inf  LinearizeAsGain=off  AntiWindupMode=none  Kb=1  POutMin=[]  POutMax=[]  IOutMin=[]  IOutMax=[]  DOutMin=[]  DOutMax=[]  NOutMin=[]  NOutMax=[]  SumOutMin=[]  SumOutMax=[]  SaturationOutMin=[]  SaturationOutMax=[]  PParamMin=[]  PParamMax=[]  IParamMin=[]  IParamMax=[]  DParamMin=[]  DParamMax=[]  NParamMin=[]  NParamMax=[]  KbParamMin=[]  KbParamMax=[]  KtParamMin=[]  KtParamMax=[]  KbOutMin=[]  KbOutMax=[]  KtOutMin=[]  KtOutMax=[]  IntegratorOutMin=[]  IntegratorOutMax=[]  FilterOutMin=[]  FilterOutMax=[]  SumI1OutMin=[]  SumI1OutMax=[]  SumI2OutMin=[]  SumI2OutMax=[]  SumI3OutMin=[]  SumI3OutMax=[]  SumI4OutMin=[]  SumI4OutMax=[]  SumDOutMin=[]  SumDOutMax=[]  DifferentiatorOutMin=[]  DifferentiatorOutMax=[]  FilterDiffOutCoefMin=[]  FilterDiffOutCoefMax=[]  ReciprocalOutMin=[]  ReciprocalOutMax=[]  SumDenOutMin=[]  SumDenOutMax=[]  SumNumOutMin=[]  SumNumOutMax=[]  DivideOutMin=[]  DivideOutMax=[]  UdiffTsProdOutMin=[]  UdiffTsProdOutMax=[]  NTsProdOutMin=[]  NTsProdOutMax=[]  UintegralTsProdOutMin=[]  UintegralTsProdOutMax=[]  UngainTsProdOutMin=[]  UngainTsProdOutMax=[]  IntegratorContinuousStateAttributes=''  IntegratorStateMustResolveToSignalObject=off  IntegratorRTWStateStorageClass=Auto  FilterContinuousStateAttributes=''  FilterStateMustResolveToSignalObject=off  FilterRTWStateStorageClass=Auto  ParallelPVariant=InternalParameters  IdealPVariant=Disabled  IVariant=InternalParameters  DVariant=InternalParameters  IntegratorVariant=Discrete  SatVariant=Disabled  AWVariant=Passthrough  PCopyVariant=Disabled  TRVariant=Disabled  FdbkBlocksVariant=Forward  IdealPFdbkVariant=Disabled  SatFdbkVariant=Disabled  DerivativeFilterVariant=ForwardEulerFilter  NVariant=InternalParameters  NCopyVariant=Disabled  FilterICVariant=InternalICsFilter  IntegratorICVariant=InternalICs  ExternalResetVariant=Disabled  TRSumVariant=Passthrough  SumFdbkVariant=Disabled  SumVariant=Sum_PID  TsampFilterVariant=InternalTs  TsampNgainVariant=Passthrough  TsampIntegralVariant=Passthrough  ExternalSaturationOutDataTypeStr=Inherit: Same as second input
  cfblk8 : Sqrt  Operator=rSqrt  OutDataTypeStr=double  AlgorithmType=Newton-Raphson  SaturateOnIntegerOverflow=on
  cfblk9 : Sum  Inputs=+-  OutDataTypeStr=double
  cyemi_{105..113} (9 alike) : DataTypeConversion  OutDataTypeStr=double
  cfblk2 : Outport
  cfblk11 : Outport  Port=2
  wires:
  cfblk9/1 -> cfblk2/1
  cfblk10/1 -> cfblk11/1
  cfblk7/1 -> cyemi_108/1, cyemi_113/1
  cyemi_105/1 -> cfblk12/1
  cfblk6/1 -> cyemi_105/1
  cyemi_106/1 -> cfblk3/1
  cfblk12/1 -> cyemi_106/1
  cyemi_107/1 -> cfblk4/1
  cfblk3/1 -> cyemi_107/1
  cyemi_108/1 -> cfblk5/1
  cyemi_109/1 -> cfblk6/1
  cfblk8/1 -> cyemi_109/1
  cyemi_110/1 -> cfblk7/1
  cfblk4/1 -> cyemi_110/1
  cyemi_111/1 -> cfblk8/1
  cfblk5/1 -> cyemi_111/1
  cyemi_112/1 -> cfblk9/1
  cfblk1/1 -> cyemi_112/1
  cyemi_113/1 -> cfblk9/2

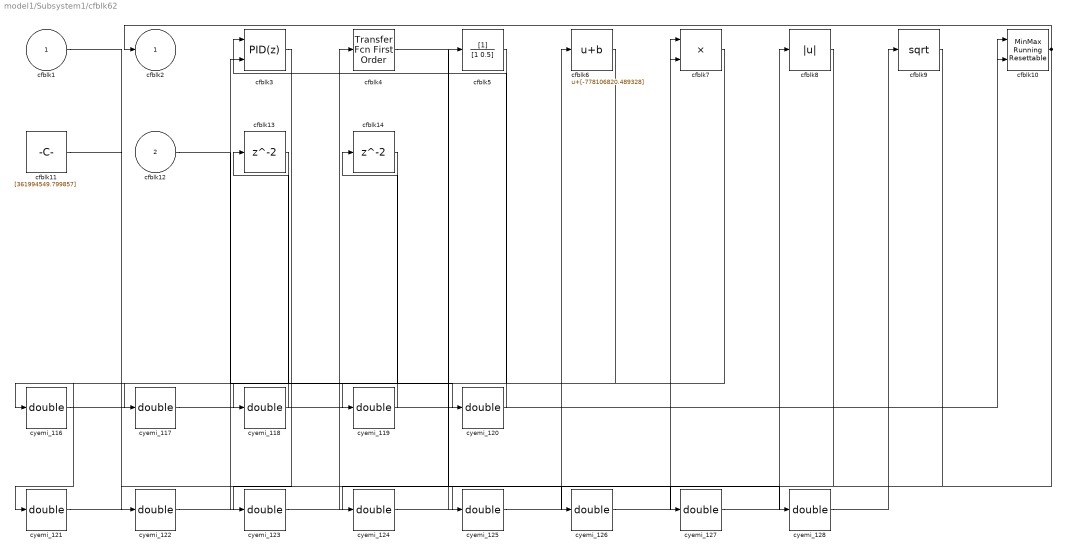
== system model1/Subsystem1/cfblk62 ==
  cfblk1 : Inport
  cfblk12 : Inport  Port=2
  cfblk10 : simulink/Math Operations/MinMax Running Resettable  Function=min  vinit=0.0
  cfblk11 : Constant  Value=[361994549.799857]  OutDataTypeStr=double  SampleTime=1
  cfblk13 : Delay  SampleTime=1
  cfblk14 : Delay  SampleTime=1
  cfblk3 : slpidlib/PID Controller (2DOF)  Controller=PID  Form=Parallel  TimeDomain=Discrete-time  UseExternalTs=off  SampleTime=1  IntegratorMethod=Forward Euler  FilterMethod=Forward Euler  ControllerParametersSource=internal  P=1  I=1  D=0  UseFilter=on  N=100  b=1  c=1  TunerSelectOption=Transfer Function Based (PID Tuner App)  InitialConditionSource=internal  InitialConditionForIntegrator=0  InitialConditionForFilter=0  DifferentiatorICPrevScaledInput=0  ExternalReset=none  TrackingMode=off  Kt=1  LimitOutput=off  SatLimitsSource=internal  UpperSaturationLimit=inf  LowerSaturationLimit=-inf  LinearizeAsGain=off  AntiWindupMode=none  Kb=1  POutMin=[]  POutMax=[]  IOutMin=[]  IOutMax=[]  DOutMin=[]  DOutMax=[]  NOutMin=[]  NOutMax=[]  bOutMin=[]  bOutMax=[]  cOutMin=[]  cOutMax=[]  SumOutMin=[]  SumOutMax=[]  SaturationOutMin=[]  SaturationOutMax=[]  PParamMin=[]  PParamMax=[]  IParamMin=[]  IParamMax=[]  DParamMin=[]  DParamMax=[]  NParamMin=[]  NParamMax=[]  bParamMin=[]  bParamMax=[]  cParamMin=[]  cParamMax=[]  KbParamMin=[]  KbParamMax=[]  KtParamMin=[]  KtParamMax=[]  KbOutMin=[]  KbOutMax=[]  KtOutMin=[]  KtOutMax=[]  IntegratorOutMin=[]  IntegratorOutMax=[]  FilterOutMin=[]  FilterOutMax=[]  SumI1OutMin=[]  SumI1OutMax=[]  SumI2OutMin=[]  SumI2OutMax=[]  SumI3OutMin=[]  SumI3OutMax=[]  SumI4OutMin=[]  SumI4OutMax=[]  SumDOutMin=[]  SumDOutMax=[]  Sum1OutMin=[]  Sum1OutMax=[]  Sum2OutMin=[]  Sum2OutMax=[]  Sum3OutMin=[]  Sum3OutMax=[]  DifferentiatorOutMin=[]  DifferentiatorOutMax=[]  FilterDiffOutCoefMin=[]  FilterDiffOutCoefMax=[]  ReciprocalOutMin=[]  ReciprocalOutMax=[]  SumDenOutMin=[]  SumDenOutMax=[]  SumNumOutMin=[]  SumNumOutMax=[]  DivideOutMin=[]  DivideOutMax=[]  UdiffTsProdOutMin=[]  UdiffTsProdOutMax=[]  NTsProdOutMin=[]  NTsProdOutMax=[]  UintegralTsProdOutMin=[]  UintegralTsProdOutMax=[]  UngainTsProdOutMin=[]  UngainTsProdOutMax=[]  IntegratorContinuousStateAttributes=''  IntegratorStateMustResolveToSignalObject=off  IntegratorRTWStateStorageClass=Auto  FilterContinuousStateAttributes=''  FilterStateMustResolveToSignalObject=off  FilterRTWStateStorageClass=Auto  ParallelPVariant=InternalParameters  IdealPVariant=Disabled  IVariant=InternalParameters  DVariant=InternalParameters  bVariant=InternalParameters  cVariant=InternalParameters  IntegratorVariant=Discrete  SatVariant=Disabled  AWVariant=Passthrough  PCopyVariant=Disabled  TRVariant=Disabled  FdbkBlocksVariant=Forward  IdealPFdbkVariant=Disabled  SatFdbkVariant=Disabled  DerivativeFilterVariant=ForwardEulerFilter  NVariant=InternalParameters  NCopyVariant=Disabled  FilterICVariant=InternalICsFilter  IntegratorICVariant=InternalICs  ExternalResetVariant=Disabled  TRSumVariant=Passthrough  SumFdbkVariant=Disabled  SumVariant=Sum_PID  TsampFilterVariant=InternalTs  TsampNgainVariant=Passthrough  TsampIntegralVariant=Passthrough  ExternalSaturationOutDataTypeStr=Inherit: Same as second input
      settings: SourceProductBaseCode=SL
  cfblk4 : simulink/Discrete/Transfer Fcn First Order  PoleZ=0.95  ICPrevOutput=0.0  DoSatur=off
  cfblk5 : DiscreteFilter  SampleTime=1
  cfblk6 : Bias  Bias=[-778106820.489328]
  cfblk7 : Product  Inputs=**  OutDataTypeStr=double
  cfblk8 : Abs  OutDataTypeStr=double
  cfblk9 : Sqrt  OutDataTypeStr=double  SaturateOnIntegerOverflow=on
  cyemi_{116..128} (13 alike) : DataTypeConversion  OutDataTypeStr=double
  cfblk2 : Outport
  wires:
  cfblk10/1 -> cfblk2/1, cyemi_124/1
  cyemi_116/1 -> cfblk10/1
  cfblk13/1 -> cyemi_116/1
  cyemi_117/1 -> cfblk10/2
  cfblk7/1 -> cyemi_117/1
  cyemi_118/1 -> cfblk13/1
  cfblk6/1 -> cyemi_118/1
  cyemi_119/1 -> cfblk14/1
  cfblk5/1 -> cyemi_119/1
  cyemi_120/1 -> cfblk3/1
  cfblk12/1 -> cyemi_120/1
  cyemi_121/1 -> cfblk3/2
  cfblk14/1 -> cyemi_121/1
  cyemi_122/1 -> cfblk4/1
  cfblk11/1 -> cyemi_122/1
  cyemi_123/1 -> cfblk5/1
  cfblk3/1 -> cyemi_123/1
  cyemi_124/1 -> cfblk6/1
  cyemi_125/1 -> cfblk7/1
  cfblk8/1 -> cyemi_125/1
  cyemi_126/1 -> cfblk7/2
  cfblk9/1 -> cyemi_126/1
  cyemi_127/1 -> cfblk8/1
  cfblk4/1 -> cyemi_127/1
  cyemi_128/1 -> cfblk9/1
  cfblk1/1 -> cyemi_128/1

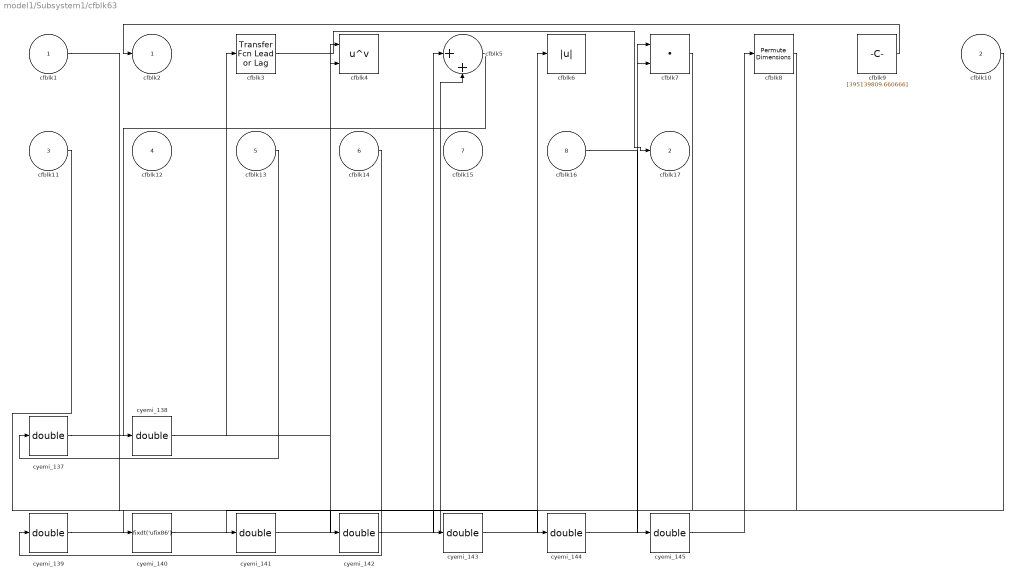
== system model1/Subsystem1/cfblk63 ==
  cfblk1 : Inport
  cfblk10 : Inport  Port=2
  cfblk11 : Inport  Port=3
  cfblk12 : Inport  Port=4
  cfblk13 : Inport  Port=5
  cfblk14 : Inport  Port=6
  cfblk15 : Inport  Port=7
  cfblk16 : Inport  Port=8
  cfblk3 : simulink/Discrete/Transfer Fcn Lead or Lag  PoleZ=0.95  ZeroZ=0.75  ICPrevOutput=0.0  ICPrevInput=0.0  DoSatur=off
      settings: SourceProductBaseCode=SL
  cfblk4 : Math  Operator=pow  OutDataTypeStr=double  SaturateOnIntegerOverflow=on
  cfblk5 : Sum  Inputs=|++  OutDataTypeStr=double
  cfblk6 : Abs  OutDataTypeStr=double
  cfblk7 : DotProduct  OutDataTypeStr=double  InputSameDT=on
  cfblk8 : PermuteDimensions
  cfblk9 : Constant  Value=[395139809.660666]  OutDataTypeStr=double  SampleTime=1
  cyemi_{137..139,141..145} (8 alike) : DataTypeConversion  OutDataTypeStr=double
  cyemi_140 : DataTypeConversion  OutDataTypeStr=fixdt('ufix86')
  cfblk2 : Outport
  cfblk17 : Outport  Port=2
  wires:
  cfblk9/1 -> cfblk2/1
  cfblk3/1 -> cfblk17/1
  cyemi_137/1 -> cfblk3/1
  cfblk13/1 -> cyemi_137/1
  cyemi_138/1 -> cfblk4/1
  cfblk5/1 -> cyemi_138/1
  cyemi_139/1 -> cfblk4/2
  cfblk14/1 -> cyemi_139/1
  cyemi_140/1 -> cfblk5/1
  cfblk11/1 -> cyemi_140/1
  cyemi_141/1 -> cfblk5/2
  cfblk10/1 -> cyemi_141/1
  cyemi_142/1 -> cfblk6/1
  cfblk7/1 -> cyemi_142/1
  cyemi_143/1 -> cfblk7/1
  cfblk8/1 -> cyemi_143/1
  cyemi_144/1 -> cfblk7/2
  cfblk1/1 -> cyemi_144/1
  cyemi_145/1 -> cfblk8/1
  cfblk16/1 -> cyemi_145/1

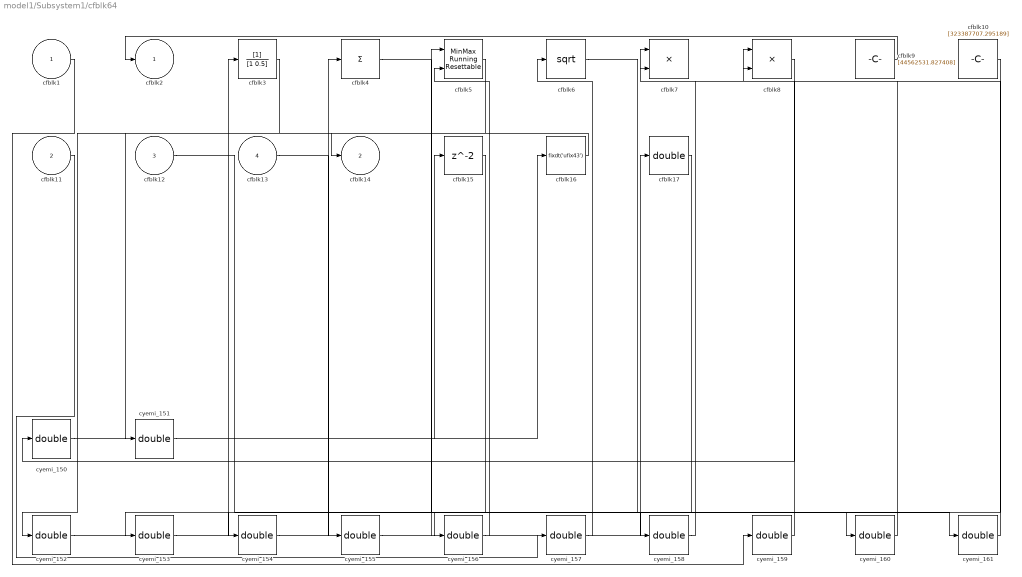
== system model1/Subsystem1/cfblk64 ==
  cfblk1 : Inport
  cfblk11 : Inport  Port=2
  cfblk12 : Inport  Port=3
  cfblk13 : Inport  Port=4
  cfblk10 : Constant  Value=[323387707.295189]  OutDataTypeStr=double  SampleTime=1
  cfblk15 : Delay  SampleTime=1
  cfblk16 : DataTypeConversion  OutDataTypeStr=fixdt('ufix43')
  cfblk17 : DataTypeConversion  OutDataTypeStr=double
  cfblk3 : DiscreteFilter  SampleTime=1
  cfblk4 : Sum  Inputs=+  OutDataTypeStr=double
  cfblk5 : simulink/Math Operations/MinMax Running Resettable  Function=min  vinit=0.0
  cfblk6 : Sqrt  OutDataTypeStr=double  SaturateOnIntegerOverflow=on
  cfblk7 : Product  Inputs=**  OutDataTypeStr=double
  cfblk8 : Product  OutDataTypeStr=double
  cfblk9 : Constant  Value=[44562531.827408]  OutDataTypeStr=double  SampleTime=1
  cyemi_{150..161} (12 alike) : DataTypeConversion  OutDataTypeStr=double
  cfblk2 : Outport
  cfblk14 : Outport  Port=2
  wires:
  cfblk9/1 -> cfblk2/1
  cfblk16/1 -> cfblk14/1
  cyemi_150/1 -> cfblk15/1
  cfblk8/1 -> cyemi_150/1
  cyemi_151/1 -> cfblk16/1
  cfblk3/1 -> cyemi_151/1
  cyemi_152/1 -> cfblk17/1
  cfblk5/1 -> cyemi_152/1
  cyemi_153/1 -> cfblk3/1
  cfblk17/1 -> cyemi_153/1
  cyemi_154/1 -> cfblk4/1
  cfblk15/1 -> cyemi_154/1
  cyemi_155/1 -> cfblk5/1
  cfblk13/1 -> cyemi_155/1
  cyemi_156/1 -> cfblk5/2
  cfblk12/1 -> cyemi_156/1
  cyemi_157/1 -> cfblk6/1
  cfblk11/1 -> cyemi_157/1
  cyemi_158/1 -> cfblk7/1
  cfblk10/1 -> cyemi_158/1
  cyemi_159/1 -> cfblk7/2
  cfblk1/1 -> cyemi_159/1
  cyemi_160/1 -> cfblk8/1
  cfblk4/1 -> cyemi_160/1
  cyemi_161/1 -> cfblk8/2
  cfblk6/1 -> cyemi_161/1

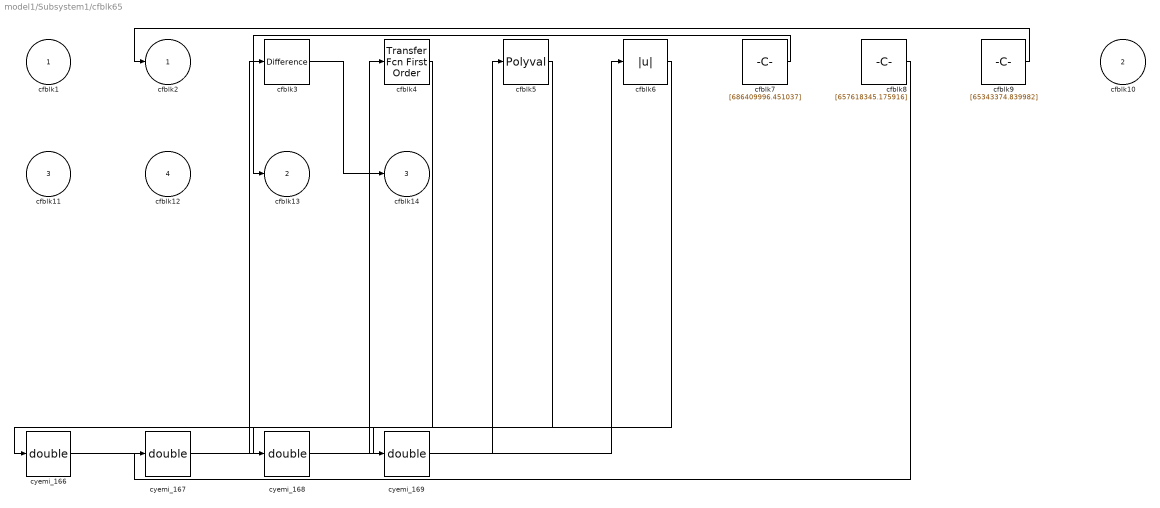
== system model1/Subsystem1/cfblk65 ==
  cfblk1 : Inport
  cfblk10 : Inport  Port=2
  cfblk11 : Inport  Port=3
  cfblk12 : Inport  Port=4
  cfblk3 : simulink/Discrete/Difference  ICPrevInput=0.0  OutMin=[]  OutMax=[]  OutDataTypeStr=double  OutputDataTypeScalingMode=double  OutDataType=fixdt(1, 16)  OutScaling=2^-10  DoSatur=off
  cfblk4 : simulink/Discrete/Transfer Fcn First Order  PoleZ=0.95  ICPrevOutput=0.0  DoSatur=off
  cfblk5 : Polyval  Coefs=[ +2.081618890e-019, -1.441693666e-014, +4.719686976e-010, -8.536869453e-006, +1.621573104e-001, -8.087801117e+001 ]
  cfblk6 : Abs  OutDataTypeStr=double
  cfblk7 : Constant  Value=[686409996.451037]  OutDataTypeStr=double  SampleTime=1
  cfblk8 : Constant  Value=[657618345.175916]  OutDataTypeStr=double  SampleTime=1
  cfblk9 : Constant  Value=[65343374.839982]  OutDataTypeStr=double  SampleTime=1
  cyemi_{166..169} (4 alike) : DataTypeConversion  OutDataTypeStr=double
  cfblk2 : Outport
  cfblk13 : Outport  Port=2
  cfblk14 : Outport  Port=3
  wires:
  cfblk3/1 -> cfblk14/1
  cfblk7/1 -> cfblk13/1
  cfblk9/1 -> cfblk2/1
  cyemi_166/1 -> cfblk3/1
  cfblk6/1 -> cyemi_166/1
  cyemi_167/1 -> cfblk4/1
  cfblk8/1 -> cyemi_167/1
  cyemi_168/1 -> cfblk5/1
  cfblk4/1 -> cyemi_168/1
  cyemi_169/1 -> cfblk6/1
  cfblk5/1 -> cyemi_169/1

== system model1/Subsystem1/cfblk66 ==
  cfblk1 : Inport
  cfblk8 : Inport  Port=2
  cfblk9 : Inport  Port=3
  cfblk3 : slpidlib/PID Controller (2DOF)  Controller=PID  Form=Parallel  TimeDomain=Discrete-time  UseExternalTs=off  SampleTime=1  IntegratorMethod=Forward Euler  FilterMethod=Forward Euler  ControllerParametersSource=internal  P=1  I=1  D=0  UseFilter=on  N=100  b=1  c=1  TunerSelectOption=Transfer Function Based (PID Tuner App)  InitialConditionSource=internal  InitialConditionForIntegrator=0  InitialConditionForFilter=0  DifferentiatorICPrevScaledInput=0  ExternalReset=none  TrackingMode=off  Kt=1  LimitOutput=off  SatLimitsSource=internal  UpperSaturationLimit=inf  LowerSaturationLimit=-inf  LinearizeAsGain=off  AntiWindupMode=none  Kb=1  POutMin=[]  POutMax=[]  IOutMin=[]  IOutMax=[]  DOutMin=[]  DOutMax=[]  NOutMin=[]  NOutMax=[]  bOutMin=[]  bOutMax=[]  cOutMin=[]  cOutMax=[]  SumOutMin=[]  SumOutMax=[]  SaturationOutMin=[]  SaturationOutMax=[]  PParamMin=[]  PParamMax=[]  IParamMin=[]  IParamMax=[]  DParamMin=[]  DParamMax=[]  NParamMin=[]  NParamMax=[]  bParamMin=[]  bParamMax=[]  cParamMin=[]  cParamMax=[]  KbParamMin=[]  KbParamMax=[]  KtParamMin=[]  KtParamMax=[]  KbOutMin=[]  KbOutMax=[]  KtOutMin=[]  KtOutMax=[]  IntegratorOutMin=[]  IntegratorOutMax=[]  FilterOutMin=[]  FilterOutMax=[]  SumI1OutMin=[]  SumI1OutMax=[]  SumI2OutMin=[]  SumI2OutMax=[]  SumI3OutMin=[]  SumI3OutMax=[]  SumI4OutMin=[]  SumI4OutMax=[]  SumDOutMin=[]  SumDOutMax=[]  Sum1OutMin=[]  Sum1OutMax=[]  Sum2OutMin=[]  Sum2OutMax=[]  Sum3OutMin=[]  Sum3OutMax=[]  DifferentiatorOutMin=[]  DifferentiatorOutMax=[]  FilterDiffOutCoefMin=[]  FilterDiffOutCoefMax=[]  ReciprocalOutMin=[]  ReciprocalOutMax=[]  SumDenOutMin=[]  SumDenOutMax=[]  SumNumOutMin=[]  SumNumOutMax=[]  DivideOutMin=[]  DivideOutMax=[]  UdiffTsProdOutMin=[]  UdiffTsProdOutMax=[]  NTsProdOutMin=[]  NTsProdOutMax=[]  UintegralTsProdOutMin=[]  UintegralTsProdOutMax=[]  UngainTsProdOutMin=[]  UngainTsProdOutMax=[]  IntegratorContinuousStateAttributes=''  IntegratorStateMustResolveToSignalObject=off  IntegratorRTWStateStorageClass=Auto  FilterContinuousStateAttributes=''  FilterStateMustResolveToSignalObject=off  FilterRTWStateStorageClass=Auto  ParallelPVariant=InternalParameters  IdealPVariant=Disabled  IVariant=InternalParameters  DVariant=InternalParameters  bVariant=InternalParameters  cVariant=InternalParameters  IntegratorVariant=Discrete  SatVariant=Disabled  AWVariant=Passthrough  PCopyVariant=Disabled  TRVariant=Disabled  FdbkBlocksVariant=Forward  IdealPFdbkVariant=Disabled  SatFdbkVariant=Disabled  DerivativeFilterVariant=ForwardEulerFilter  NVariant=InternalParameters  NCopyVariant=Disabled  FilterICVariant=InternalICsFilter  IntegratorICVariant=InternalICs  ExternalResetVariant=Disabled  TRSumVariant=Passthrough  SumFdbkVariant=Disabled  SumVariant=Sum_PID  TsampFilterVariant=InternalTs  TsampNgainVariant=Passthrough  TsampIntegralVariant=Passthrough  ExternalSaturationOutDataTypeStr=Inherit: Same as second input
      settings: SourceProductBaseCode=SL
  cfblk4 : Sqrt  OutDataTypeStr=double  SaturateOnIntegerOverflow=on
  cfblk5 : Assignment  DiagnosticForDimensions=Warning  IndexOptions=Index vector (dialog)  Indices=1  OutputSizes=1
  cfblk6 : Constant  Value=[-723852700.126634]  OutDataTypeStr=double  SampleTime=1
  cfblk7 : Constant  Value=[458252857.002176]  OutDataTypeStr=double  SampleTime=1
  cyemi_{173..177} (5 alike) : DataTypeConversion  OutDataTypeStr=double
  cfblk2 : Outport
  wires:
  cfblk5/1 -> cfblk2/1
  cyemi_173/1 -> cfblk3/1
  cfblk6/1 -> cyemi_173/1
  cyemi_174/1 -> cfblk3/2
  cfblk7/1 -> cyemi_174/1
  cyemi_175/1 -> cfblk4/1
  cfblk1/1 -> cyemi_175/1
  cyemi_176/1 -> cfblk5/1
  cfblk9/1 -> cyemi_176/1
  cyemi_177/1 -> cfblk5/2
  cfblk3/1 -> cyemi_177/1

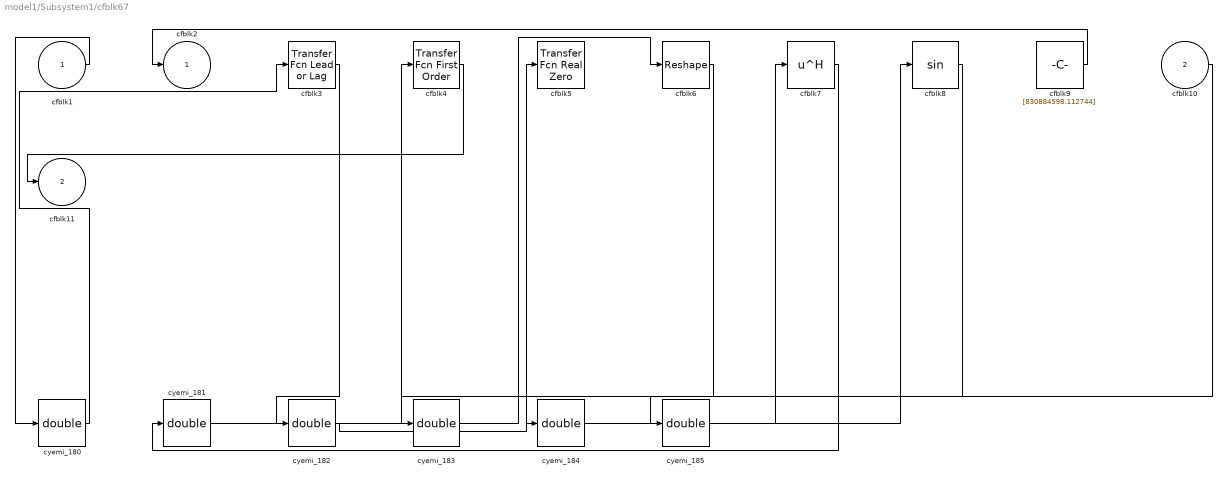
== system model1/Subsystem1/cfblk67 ==
  cfblk1 : Inport
  cfblk10 : Inport  Port=2
  cfblk3 : simulink/Discrete/Transfer Fcn Lead or Lag  PoleZ=0.95  ZeroZ=0.75  ICPrevOutput=0.0  ICPrevInput=0.0  DoSatur=off
      settings: SourceProductBaseCode=SL
  cfblk4 : simulink/Discrete/Transfer Fcn First Order  PoleZ=0.95  ICPrevOutput=0.0  DoSatur=off
  cfblk5 : simulink/Discrete/Transfer Fcn Real Zero  ZeroZ=0.75  ICPrevInput=0.0  DoSatur=off
      settings: SourceProductBaseCode=SL
  cfblk6 : Reshape
  cfblk7 : Math  Operator=hermitian  OutDataTypeStr=double  SaturateOnIntegerOverflow=on
  cfblk8 : Trigonometry
  cfblk9 : Constant  Value=[830884598.112744]  OutDataTypeStr=double  SampleTime=1
  cyemi_{180..185} (6 alike) : DataTypeConversion  OutDataTypeStr=double
  cfblk2 : Outport
  cfblk11 : Outport  Port=2
  wires:
  cfblk4/1 -> cfblk11/1
  cfblk9/1 -> cfblk2/1
  cyemi_180/1 -> cfblk3/1
  cfblk1/1 -> cyemi_180/1
  cyemi_181/1 -> cfblk4/1
  cfblk7/1 -> cyemi_181/1
  cyemi_182/1 -> cfblk5/1
  cfblk3/1 -> cyemi_182/1
  cyemi_183/1 -> cfblk6/1
  cfblk8/1 -> cyemi_183/1
  cyemi_184/1 -> cfblk7/1
  cfblk6/1 -> cyemi_184/1
  cyemi_185/1 -> cfblk8/1
  cfblk10/1 -> cyemi_185/1
